simulink library "prelab1Library"  (R2020a)
settings: Solver=VariableStepAuto  StartTime=0.0  StopTime=10.0  RelTol=1e-3
settings Model: Creator=brucecui  LastModifiedBy=brucecui

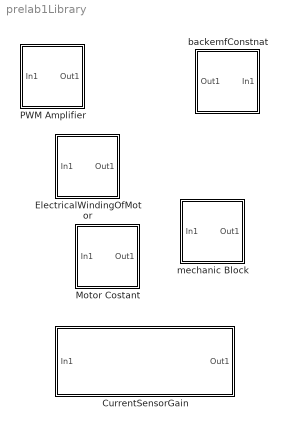
== system prelab1Library ==
  CurrentSensorGain : Subsystem
  ElectricalWindingOfMotor : Subsystem
  Motor Costant : Subsystem
  PWM Amplifier : Subsystem
  backemfConstnat : Subsystem
  mechanic Block : Subsystem

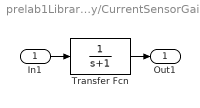
== system prelab1Library/CurrentSensorGain ==
  In1 : Inport
  Transfer Fcn : TransferFcn  Denominator=[1 1]
  Out1 : Outport
  wires:
  In1/1 -> Transfer Fcn/1
  Transfer Fcn/1 -> Out1/1

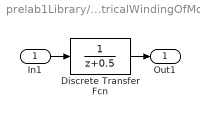
== system prelab1Library/ElectricalWindingOfMotor ==
  In1 : Inport
  Discrete Transfer Fcn : DiscreteTransferFcn
  Out1 : Outport
  wires:
  In1/1 -> Discrete Transfer Fcn/1
  Discrete Transfer Fcn/1 -> Out1/1

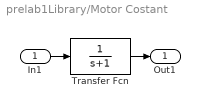
== system prelab1Library/Motor Costant ==
  In1 : Inport
  Transfer Fcn : TransferFcn  Denominator=[1 1]
  Out1 : Outport
  wires:
  Transfer Fcn/1 -> Out1/1
  In1/1 -> Transfer Fcn/1

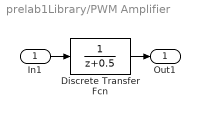
== system prelab1Library/PWM Amplifier ==
  In1 : Inport
  Discrete Transfer Fcn : DiscreteTransferFcn
  Out1 : Outport
  wires:
  Discrete Transfer Fcn/1 -> Out1/1
  In1/1 -> Discrete Transfer Fcn/1

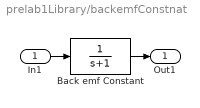
== system prelab1Library/backemfConstnat ==
  In1 : Inport
  Back emf Constant : TransferFcn  Denominator=[1 1]
  Out1 : Outport
  wires:
  Back emf Constant/1 -> Out1/1
  In1/1 -> Back emf Constant/1

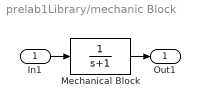
== system prelab1Library/mechanic Block ==
  In1 : Inport
  Mechanical Block : TransferFcn  Denominator=[1 1]
  Out1 : Outport
  wires:
  In1/1 -> Mechanical Block/1
  Mechanical Block/1 -> Out1/1
